simulink model "pendulam"  (R2023a)
settings: Solver=VariableStepAuto  StartTime=0.0  StopTime=10.0  MaxStep=0.01  RelTol=1e-3
undefined symbols (not defined in the file): beta, g, l, m
settings Model: Creator=agraw  LastModifiedBy=agraw

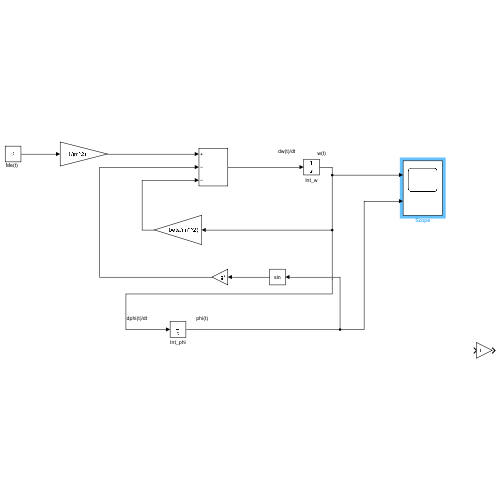
[thumbnail: Simulink's stored preview of the top-level diagram]
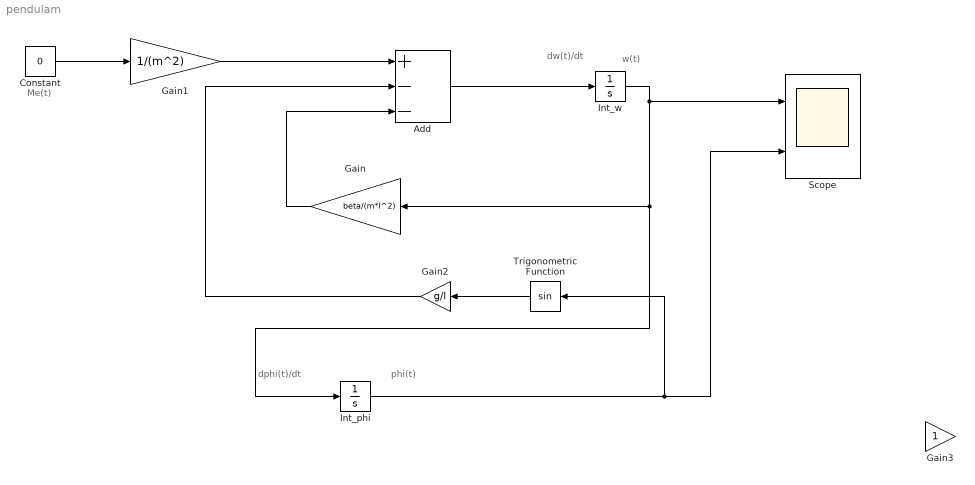
== system pendulam ==
  note: Me(t)
  note: dphi(t)/dt
  note: phi(t)
  note: dw(t)/dt
  note: w(t)
  Add : Sum  Inputs=+--
  Constant : Constant  Value=0
  Gain : Gain  Gain=beta/(m*l^2)
  Gain1 : Gain  Gain=1/(m^2)
  Gain2 : Gain  Gain=g/l
  Gain3 : Gain
  Int_phi : Integrator  InitialCondition=pi*0.999
  Int_w : Integrator
  Scope : Scope  NumInputPorts=2
  Trigonometric Function : Trigonometry
  wires:
  Int_w/1 -> Scope/1, Int_phi/1, Gain/1
  Add/1 -> Int_w/1
  Gain/1 -> Add/3
  Int_phi/1 -> Scope/2, Trigonometric Function/1
  Trigonometric Function/1 -> Gain2/1
  Gain2/1 -> Add/2
  Gain1/1 -> Add/1
  Constant/1 -> Gain1/1
